simulink model "Deliverable1_3K04"  (R2023b)
settings: Solver=VariableStepAuto  StartTime=0.0  StopTime=10.0  RelTol=1e-3
undefined symbols (not defined in the file): D0, D1, D10, D11, D12, D13, D2, D3, D4, D5, D6, D7, D8, D9, PTA0, PTA1, PTA2, PTB23, PTB9, PTC16, PTC17, PTC2, PTC3, PTC4, PTD0, PTD1, PTD2, PTD3
libraries: frdmk64flib x14
settings Model: Creator=reemb  LastModifiedBy=reemb

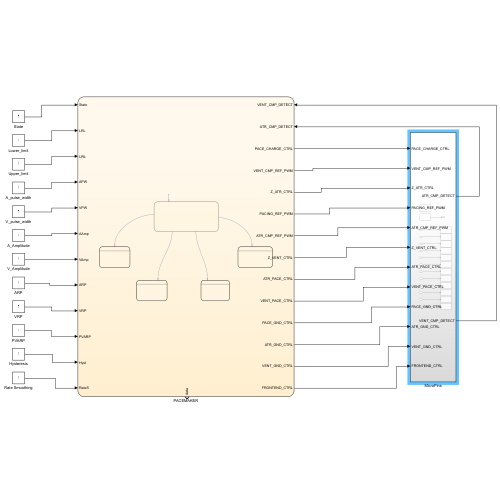
[thumbnail: Simulink's stored preview of the top-level diagram]
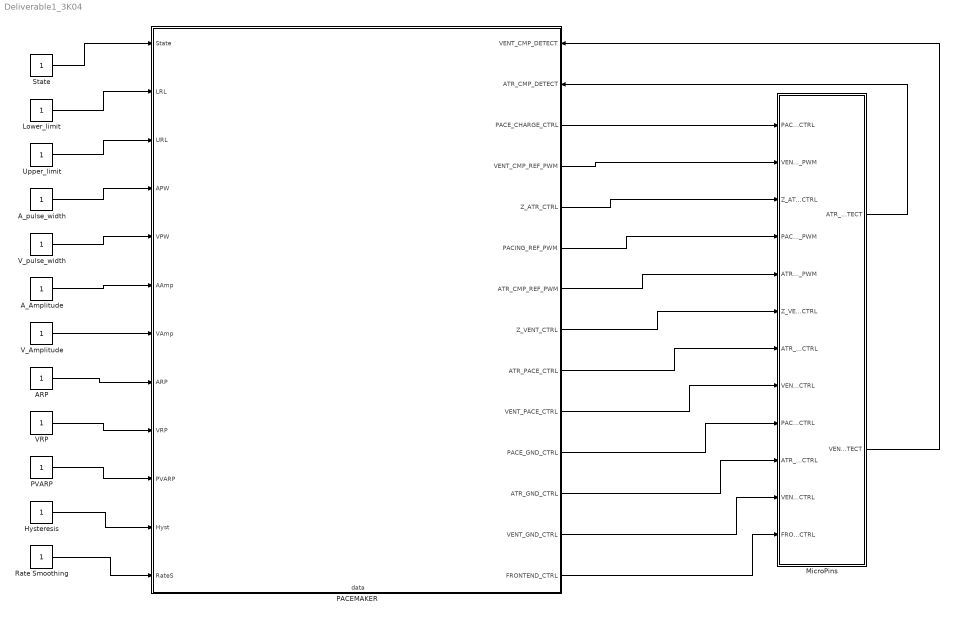
== system Deliverable1_3K04 ==
  ARP : Constant
  A_Amplitude : Constant
  A_pulse_width : Constant
  Hysteresis : Constant
  Lower_limit : Constant
  MicroPins : Subsystem
  PACEMAKER : Stateflow chart  TreatAsAtomicUnit=on
      settings: PortSchema="{\"entries\":[{\"content\":{\"sides\":[{\"content\":{\"connectorIds\":[\"In3\",\"In4\",\"In5\",\"In6\",\"In7\",\"In8\",\"In9\",\"In10\",\"In11\",\"In12\",\"In13\",\"In14\"]},\"type\":\"ConnectorPlacement.EquallySpacedRectSide\",\"uuid\":\"7cbba28d-d6b5-400e-9a50-b0e37a8211d4\"},{\"content\":{\"connectorIds\":[\"In1\",\"In2\",\"Out2\",\"Out3\",\"Out4\",\"Out5\",\"Out6\",\"Out7\",\"Out8\",\"Out9\",\"Out10\",\"Out11\",\"Out12\",\"Out13\"],\"side\":\"RIGHT\"},\"type\":\"ConnectorPlacement.EquallySpacedRectSide\",\"uuid\":\"2a786561-2bcf-4c7f-b8b6-f891341fddbf\"},{\"content\":{\"side\":\"TOP\"},\"type\":\"ConnectorPlacement.EquallySpacedRectSide\",\"uuid\":\"7b6f461d-3b2d-4b32-9979-f521bc7d7c1b\"},{\"content\":{\"connectorIds\":[\"Out1\"],\"side\":\"BOTTOM\"},\"type\":\"ConnectorPlacement.EquallySpacedRectSide\",\"uuid\":\"770127f9-5f58-4f6b-a29d-753cbd1f482a\"}]},\"type\":\"ConnectorPlacement.EquallySpacedConnector\",\"uuid\":\"c647d80e-c044-49f8-bb98-b0e1d3dd5325\"}],\"packageUris\":[\"http://schema.mathworks.com/mf0/Connector/R2020b\"],\"version\":\"1.0\"}"
  PVARP : Constant
  Rate Smoothing : Constant
  State : Constant
  Upper_limit : Constant
  VRP : Constant
  V_Amplitude : Constant
  V_pulse_width : Constant
  wires:
  State/1 -> PACEMAKER/3(State)
  Upper_limit/1 -> PACEMAKER/5(URL)
  A_Amplitude/1 -> PACEMAKER/8(AAmp)
  ARP/1 -> PACEMAKER/10(ARP)
  VRP/1 -> PACEMAKER/11(VRP)
  Hysteresis/1 -> PACEMAKER/13(Hyst)
  PVARP/1 -> PACEMAKER/12(PVARP)
  Lower_limit/1 -> PACEMAKER/4(LRL)
  V_Amplitude/1 -> PACEMAKER/9(VAmp)
  Rate Smoothing/1 -> PACEMAKER/14(RateS)
  V_pulse_width/1 -> PACEMAKER/7(VPW)
  A_pulse_width/1 -> PACEMAKER/6(APW)
  PACEMAKER/12(VENT_GND_CTRL) -> MicroPins/11(VENT_GND_CTRL)
  PACEMAKER/7(Z_VENT_CTRL) -> MicroPins/6(Z_VENT_CTRL)
  PACEMAKER/6(ATR_CMP_REF_PWM) -> MicroPins/5(ATR_CMP_REF_PWM)
  PACEMAKER/4(Z_ATR_CTRL) -> MicroPins/3(Z_ATR_CTRL)
  PACEMAKER/2(PACE_CHARGE_CTRL) -> MicroPins/1(PACE_CHARGE_CTRL)
  PACEMAKER/3(VENT_CMP_REF_PWM) -> MicroPins/2(VENT_CMP_REF_PWM)
  PACEMAKER/5(PACING_REF_PWM) -> MicroPins/4(PACING_REF_PWM)
  PACEMAKER/11(ATR_GND_CTRL) -> MicroPins/10(ATR_GND_CTRL)
  PACEMAKER/10(PACE_GND_CTRL) -> MicroPins/9(PACE_GND_CTRL)
  PACEMAKER/8(ATR_PACE_CTRL) -> MicroPins/7(ATR_PACE_CTRL)
  PACEMAKER/9(VENT_PACE_CTRL) -> MicroPins/8(VENT_PACE_CTRL)
  PACEMAKER/13(FRONTEND_CTRL) -> MicroPins/12(FRONTEND_CTRL)
  MicroPins/1(ATR_CMP_DETECT) -> PACEMAKER/2(ATR_CMP_DETECT)
  MicroPins/2(VENT_CMP_DETECT) -> PACEMAKER/1(VENT_CMP_DETECT)

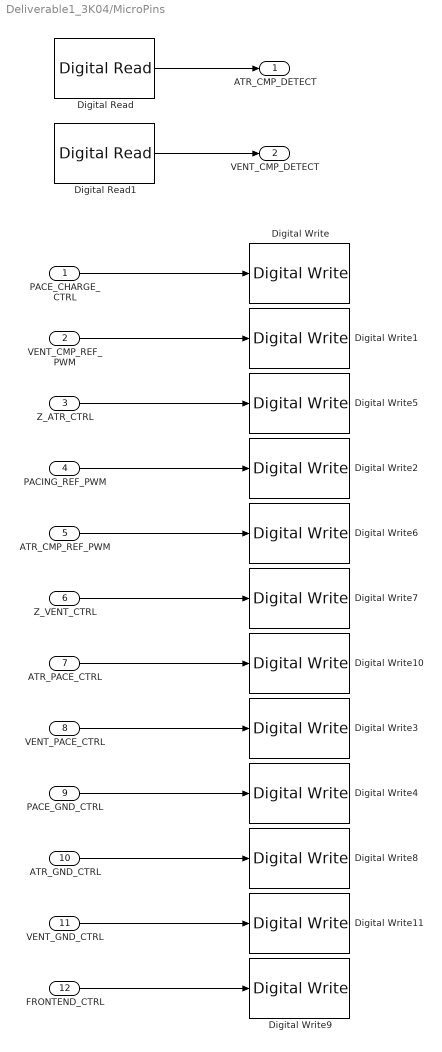
== system Deliverable1_3K04/MicroPins ==
  PACE_CHARGE_CTRL : Inport
  VENT_CMP_REF_PWM : Inport  Port=2
  Z_ATR_CTRL : Inport  Port=3
  PACING_REF_PWM : Inport  Port=4
  ATR_CMP_REF_PWM : Inport  Port=5
  Z_VENT_CTRL : Inport  Port=6
  ATR_PACE_CTRL : Inport  Port=7
  VENT_PACE_CTRL : Inport  Port=8
  PACE_GND_CTRL : Inport  Port=9
  ATR_GND_CTRL : Inport  Port=10
  VENT_GND_CTRL : Inport  Port=11
  FRONTEND_CTRL : Inport  Port=12
  Digital Read : frdmk64flib/Digital Read  Whichpin=PTC16 (D0)  SampleTime=-1
  Digital Read1 : frdmk64flib/Digital Read  Whichpin=PTC17 (D1)  SampleTime=-1
  Digital Write : frdmk64flib/Digital Write  Whichpin=PTB9 (D2)
  Digital Write1 : frdmk64flib/Digital Write  Whichpin=PTA1 (D3)
  Digital Write10 : frdmk64flib/Digital Write  Whichpin=PTA0 (D8)
  Digital Write11 : frdmk64flib/Digital Write  Whichpin=PTD3 (D12)
  Digital Write2 : frdmk64flib/Digital Write  Whichpin=PTA2 (D5)
  Digital Write3 : frdmk64flib/Digital Write  Whichpin=PTC4 (D9)
  Digital Write4 : frdmk64flib/Digital Write  Whichpin=PTD0 (D10)
  Digital Write5 : frdmk64flib/Digital Write  Whichpin=PTB23 (D4)
  Digital Write6 : frdmk64flib/Digital Write  Whichpin=PTC2 (D6)
  Digital Write7 : frdmk64flib/Digital Write  Whichpin=PTC3 (D7)
  Digital Write8 : frdmk64flib/Digital Write  Whichpin=PTD2 (D11)
  Digital Write9 : frdmk64flib/Digital Write  Whichpin=PTD1 (D13)
  ATR_CMP_DETECT : Outport
  VENT_CMP_DETECT : Outport  Port=2
  wires:
  Digital Read/1 -> ATR_CMP_DETECT/1
  Digital Read1/1 -> VENT_CMP_DETECT/1
  PACE_CHARGE_CTRL/1 -> Digital Write/1
  FRONTEND_CTRL/1 -> Digital Write9/1
  VENT_GND_CTRL/1 -> Digital Write11/1
  ATR_GND_CTRL/1 -> Digital Write8/1
  PACE_GND_CTRL/1 -> Digital Write4/1
  VENT_PACE_CTRL/1 -> Digital Write3/1
  ATR_PACE_CTRL/1 -> Digital Write10/1
  Z_VENT_CTRL/1 -> Digital Write7/1
  ATR_CMP_REF_PWM/1 -> Digital Write6/1
  PACING_REF_PWM/1 -> Digital Write2/1
  Z_ATR_CTRL/1 -> Digital Write5/1
  VENT_CMP_REF_PWM/1 -> Digital Write1/1

== stateflow chart Deliverable1_3K04/PACEMAKER ==
  state InitalState
  state AOO
    state Charging_Discharging
      %discharge
      ATR_GND_CTRL = 1;
      PACE_GND_CTRL = 0;
      ATR_PACE_CTRL = 0;
      VENT_PACE_CTRL = 0;
      VENT_GND_CTRL = 0;
      Z_ATR_CTRL =0;
      Z_VENT_CTRL = 0;
      LED_ON = 0;
      %charge
      PACE_CHARGE_CTRL =1;
      ATR_PACE_CTRL =0;
      VENT_PACE_CTRL = 0;
      PACING_REF_PWM = A_Amplitude; %math, need desired duty cycle
    state Pacing
      PACE_GND_CTRL = 1;
      ATR_PACE_CTRL = 1;
      PACE_CHARGE_CTRL = 0;
      ATR_GND_CTRL = 0;
      VENT_PACE_CTRL = 0;
      VENT_GND_CTRL = 0;
      Z_ATR_CTRL = 0;
      Z_VENT_CTRL = 0;
    (default) -> AOO.Charging_Discharging
    AOO.Charging_Discharging -> AOO.Pacing : [after(Lower_limit - A_pulse_width, msec)]
    AOO.Pacing -> AOO.Charging_Discharging : [after(A_pulse_width, msec)]
  state VVI
  state VOO
    state Pacing
      PACE_GND_CTRL = 1;
      VENT_PACE_CTRL = 1;
      PACE_CHARGE_CTRL = 0;
      ATR_PACE_CTRL = 0;
      ATR_GND_CTRL = 0;
      VENT_GND_CTRL = 0;
      Z_ATR_CTRL = 0;
      Z_VENT_CTRL = 0;
    state Charging_Discharging
      %discharging
      PACE_GND_CTRL = 1;
      VENT_GND_CTRL = 1;
      ATR_PACE_CTRL = 0;
      ATR_GND_CTRL = 0;
      VENT_PACE_CTRL = 0;
      Z_ATR_CTRL = 0;
      Z_VENT_CTRL = 0;
      %charging
      PACE_CHARGE_CTRL = 1;
      ATR_PACE_CTRL = 0;
      VENT_PACE_CTRL = 0;
      PACING_REF_PWM = V_Amplitude %math
    (default) -> VOO.Charging_Discharging
    VOO.Charging_Discharging -> VOO.Pacing : [after(Lower_limit - V_pulse_width, msec)]
    VOO.Pacing -> VOO.Charging_Discharging : [after(V_pulse_width, msec)]
  state AAI
  (default) -> InitalState
  InitalState -> AOO [order 1] : [State == 1]
  InitalState -> VVI [order 4] : [State == 4]
  InitalState -> VOO [order 2] : [State == 2]
  InitalState -> AAI [order 3] : [State == 3]
  data: data output; VENT_CMP_DETECT input; ATR_CMP_DETECT input; PACE_CHARGE_CTRL output; VENT_CMP_REF_PWM output; Z_ATR_CTRL output; PACING_REF_PWM output; ATR_CMP_REF_PWM output; Z_VENT_CTRL output; ATR_PACE_CTRL output; VENT_PACE_CTRL output; PACE_GND_CTRL output; ATR_GND_CTRL output; State input; LRL input; URL input; APW input; VPW input; AAmp input; VAmp input; ARP input; VRP input; PVARP input; Hyst input; RateS input; VENT_GND_CTRL output; FRONTEND_CTRL output
